simulink model "DBPSK_FormaEficiente"  (R2018b)
settings: Solver=ode5  StartTime=0.0  StopTime=(1/Rb)*CantSimb  FixedStep=(1/Rb)/1000  RelTol=1e-3
values from neighbouring files (symbols this model uses):
  Eb = EbPerf    [BDPSK.m]    (also in Codigo8DPSK.m; CodigoQDPSK.m)
  Fp = 10*Rb    [BDPSK.m]    (also in Codigo8DPSK.m; CodigoQDPSK.m)
  Rb = RbPerf    [BDPSK.m]    (also in Codigo8DPSK.m; CodigoQDPSK.m)
libraries: dspsigops x3, simulink x2, commchan3 x1, commrandsrc3 x1, commdigbbndpm3 x1
settings Model: Creator=lukit  LastModifiedBy=lukit

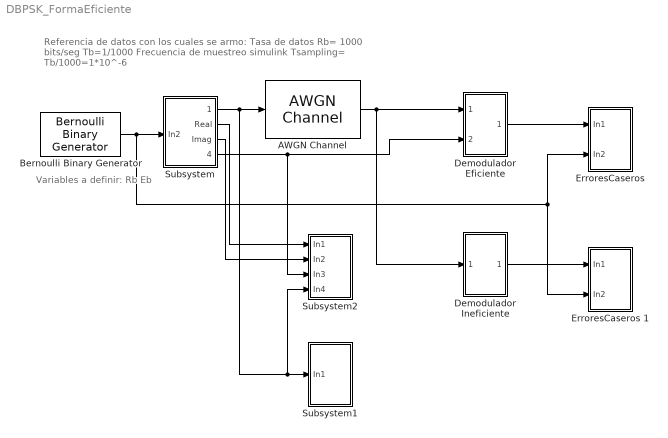
== system DBPSK_FormaEficiente ==
  note: Variables a definir:
      | Rb
      | Eb
  note: Referencia de datos con los cuales se armo:
      | Tasa de datos Rb= 1000 bits/seg Tb=1/1000
      | Frecuencia de muestreo simulink Tsampling= Tb/1000=1*10^-6
  AWGN Channel : commchan3/AWGN Channel  InputProcessing=Columns as channels (frame based)  seed=67  noiseMode="Signal to noise ratio  (Es/No)"  EbNodB=EsNo  EsNodB=EsNo  SNRdB=2  bitsPerSym=1  Ps=Eb/(1/Rb)  Tsym=(1/Rb)  variance=1
      settings: SourceProductName=Communications Toolbox
  Bernoulli Binary Generator : commrandsrc3/Bernoulli Binary Generator  ProbabilityOfZero=0.5  SeedSource=Auto  Seed=0  SampleTime=1/Rb  SamplesPerFrame=1  OutputDataType=double  SimulateUsing=Interpreted execution
      settings: SourceProductName=Communications Toolbox
  Demodulador Eficiente : Subsystem
  "Demodulador Ineficiente " : Subsystem
  "ErroresCaseros " : Subsystem
  ErroresCaseros 1 : Subsystem
  Subsystem : Subsystem
  Subsystem1 : Subsystem
  Subsystem2 : Subsystem
  wires:
  Bernoulli Binary Generator/1 -> ErroresCaseros 1/2(In2), "ErroresCaseros "/2(In2), Subsystem/1(In2)
  Subsystem/1(Salida) -> Subsystem2/4(In4), Subsystem1/1(In1), AWGN Channel/1
  Subsystem/4("Secuencia ") -> Subsystem2/3(In3), Demodulador Eficiente/2(In2)
  Demodulador Eficiente/1(Out1) -> "ErroresCaseros "/1(In1)
  AWGN Channel/1 -> "Demodulador Ineficiente "/1(In1), Demodulador Eficiente/1(In1)
  "Demodulador Ineficiente "/1(Out1) -> ErroresCaseros 1/1(In1)
  Subsystem/2(Real) -> Subsystem2/1(In1)
  Subsystem/3(Imag) -> Subsystem2/2(In2)

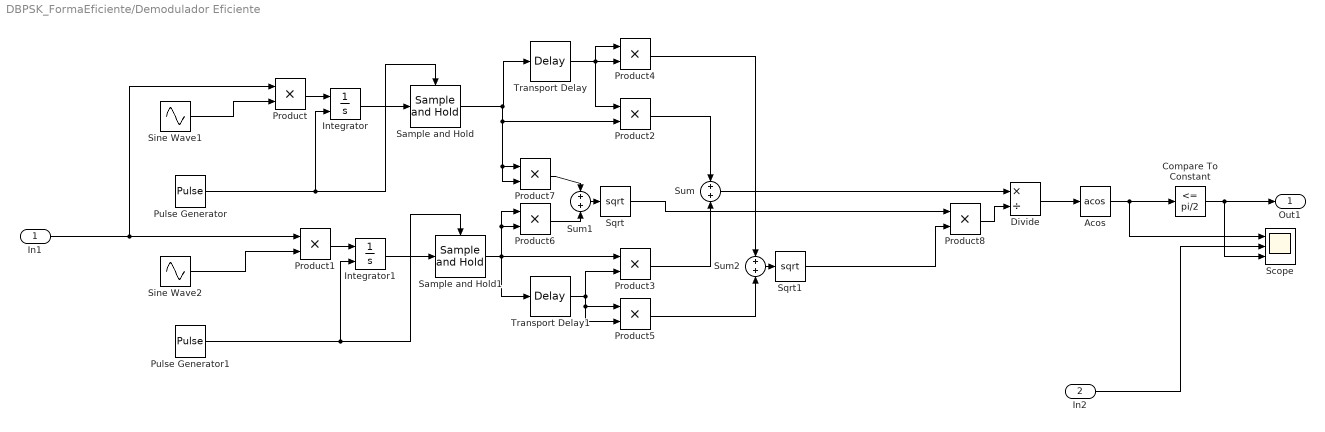
== system DBPSK_FormaEficiente/Demodulador Eficiente ==
  In1 : Inport
  In2 : Inport  Port=2
  Acos : Trigonometry  Operator=acos
  Compare To Constant : simulink/Logic and Bit Operations/Compare To Constant  relop=<=  const=pi/2  OutDataTypeStr=boolean
  Divide : Product  Inputs=*/
  Integrator : Integrator  ExternalReset=rising
  Integrator1 : Integrator  ExternalReset=rising
  Product{,1..8} (9 alike) : Product
  Pulse Generator : DiscretePulseGenerator  PulseType=Time based  Period=1/Rb  PulseWidth=99
  Pulse Generator1 : DiscretePulseGenerator  PulseType=Time based  Period=1/Rb  PulseWidth=99
  Sample and Hold : dspsigops/Sample and Hold  trig=Falling edge  initCond=0  latchinput=off
  Sample and Hold1 : dspsigops/Sample and Hold  trig=Falling edge  initCond=0  latchinput=off
  Scope : Scope  NumInputPorts=3
  Sine Wave1 : Sin  Amplitude=sqrt(2/(1/Rb))  Frequency=2*pi*Fp  Phase=pi/2
  Sine Wave2 : Sin  Amplitude=sqrt(2/(1/Rb))  Frequency=2*pi*Fp
  Sqrt : Sqrt  SaturateOnIntegerOverflow=on
  Sqrt1 : Sqrt  SaturateOnIntegerOverflow=on
  Sum : Sum
  Sum1 : Sum
  Sum2 : Sum
  Transport Delay : TransportDelay  DelayTime=1/Rb
  Transport Delay1 : TransportDelay  DelayTime=1/Rb
  Out1 : Outport
  wires:
  Integrator/1 -> Sample and Hold/1
  Pulse Generator/1 -> Sample and Hold/Trigger, Integrator/2
  Product/1 -> Integrator/1
  Integrator1/1 -> Sample and Hold1/1
  Product1/1 -> Integrator1/1
  Pulse Generator1/1 -> Sample and Hold1/Trigger, Integrator1/2
  Sample and Hold/1 -> Product7/2, Product7/1, Product2/2, Transport Delay/1
  Sample and Hold1/1 -> Product6/2, Product6/1, Transport Delay1/1, Product3/1
  Transport Delay1/1 -> Product5/2, Product5/1, Product3/2
  Transport Delay/1 -> Product4/1, Product4/2, Product2/1
  Product2/1 -> Sum/1
  Product3/1 -> Sum/2
  Product7/1 -> Sum1/1
  Product6/1 -> Sum1/2
  Sum1/1 -> Sqrt/1
  Product5/1 -> Sum2/2
  Product4/1 -> Sum2/1
  Sum2/1 -> Sqrt1/1
  Sum/1 -> Divide/1
  Product8/1 -> Divide/2
  Sqrt1/1 -> Product8/2
  Sqrt/1 -> Product8/1
  Divide/1 -> Acos/1
  Sine Wave1/1 -> Product/2
  Sine Wave2/1 -> Product1/2
  Acos/1 -> Compare To Constant/1, Scope/1
  In1/1 -> Product1/1, Product/1
  In2/1 -> Scope/2
  Compare To Constant/1 -> Scope/3, Out1/1

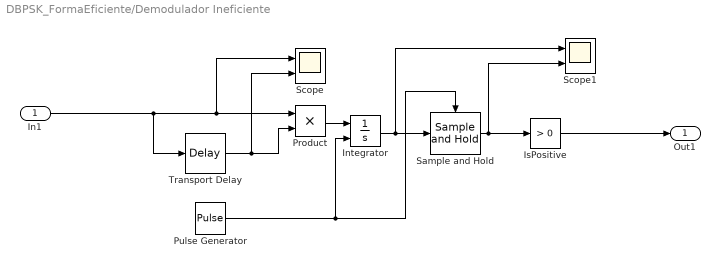
== system DBPSK_FormaEficiente/Demodulador Ineficiente  ==
  In1 : Inport
  Integrator : Integrator  ExternalReset=rising
  IsPositive : simulink/Logic and Bit Operations/Compare To Zero  relop=>  OutDataTypeStr=boolean
  Product : Product
  Pulse Generator : DiscretePulseGenerator  PulseType=Time based  Period=1/Rb  PulseWidth=99
  Sample and Hold : dspsigops/Sample and Hold  trig=Falling edge  initCond=0  latchinput=off
  Scope : Scope  NumInputPorts=2
  Scope1 : Scope  NumInputPorts=2
  Transport Delay : TransportDelay  DelayTime=(1/Rb)
  Out1 : Outport
  wires:
  Sample and Hold/1 -> Scope1/2, IsPositive/1
  In1/1 -> Transport Delay/1, Scope/1, Product/1
  Transport Delay/1 -> Product/2, Scope/2
  Integrator/1 -> Scope1/1, Sample and Hold/1
  Pulse Generator/1 -> Sample and Hold/Trigger, Integrator/2
  Product/1 -> Integrator/1
  IsPositive/1 -> Out1/1

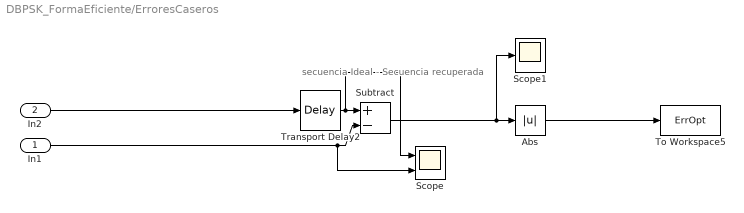
== system DBPSK_FormaEficiente/ErroresCaseros  ==
  note: secuencia Ideal - Secuencia recuperada
  In1 : Inport
  In2 : Inport  Port=2
  Abs : Abs
  Scope : Scope  NumInputPorts=2
  Scope1 : Scope
  Subtract : Sum  Inputs=+-
  To Workspace5 : ToWorkspace  VariableName=ErrOpt  SampleTime=-1
      settings: Save2DSignal=2-D array (concatenate along first dimension)
  Transport Delay2 : TransportDelay  DelayTime=(1/Rb)
  wires:
  Subtract/1 -> Scope1/1, Abs/1
  Transport Delay2/1 -> Scope/1, Subtract/1
  In1/1 -> Scope/2, Subtract/2
  In2/1 -> Transport Delay2/1
  Abs/1 -> To Workspace5/1

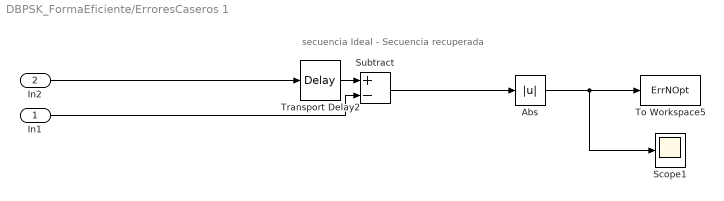
== system DBPSK_FormaEficiente/ErroresCaseros 1 ==
  note: secuencia Ideal - Secuencia recuperada
  In1 : Inport
  In2 : Inport  Port=2
  Abs : Abs
  Scope1 : Scope
  Subtract : Sum  Inputs=+-
  To Workspace5 : ToWorkspace  VariableName=ErrNOpt  SampleTime=-1
      settings: Save2DSignal=2-D array (concatenate along first dimension)
  Transport Delay2 : TransportDelay  DelayTime=(1/Rb)
  wires:
  Transport Delay2/1 -> Subtract/1
  In1/1 -> Subtract/2
  In2/1 -> Transport Delay2/1
  Subtract/1 -> Abs/1
  Abs/1 -> Scope1/1, To Workspace5/1

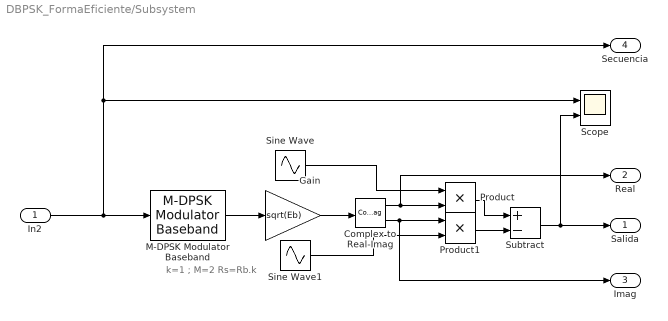
== system DBPSK_FormaEficiente/Subsystem ==
  note: k=1 ; M=2
      | Rs=Rb.k
  In2 : Inport
  Complex to Real-Imag : ComplexToRealImag
  Gain : Gain  Gain=sqrt(Eb)
  M-DPSK Modulator Baseband : commdigbbndpm3/M-DPSK Modulator Baseband  M=2  InType=Bit  Enc=Binary  Ph=pi  outDtype=double
      settings: SourceProductName=Communications Toolbox  SourceProductBaseCode=CM
  Product : Product
  Product1 : Product
  Scope : Scope  NumInputPorts=2
  Sine Wave : Sin  Amplitude=sqrt(2/(1/Rb))  Frequency=2*pi*Fp  Phase=pi/2
  Sine Wave1 : Sin  Amplitude=sqrt(2/(1/Rb))  Frequency=2*pi*Fp
  Subtract : Sum  Inputs=+-
  Salida : Outport
  Real : Outport  Port=2
  Imag : Outport  Port=3
  "Secuencia " : Outport  Port=4
  wires:
  Product/1 -> Subtract/1
  M-DPSK Modulator Baseband/1 -> Gain/1
  Sine Wave1/1 -> Product1/2
  Product1/1 -> Subtract/2
  Complex to Real-Imag/2 -> Imag/1, Product1/1
  Sine Wave/1 -> Product/1
  Complex to Real-Imag/1 -> Product/2, Real/1
  Subtract/1 -> Salida/1, Scope/2
  Gain/1 -> Complex to Real-Imag/1
  In2/1 -> M-DPSK Modulator Baseband/1, Scope/1, "Secuencia "/1

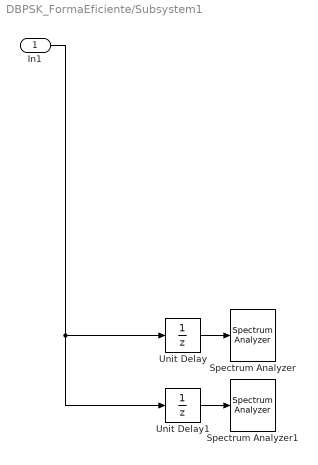
== system DBPSK_FormaEficiente/Subsystem1 ==
  In1 : Inport
  Spectrum Analyzer : SpectrumAnalyzer
  Spectrum Analyzer1 : SpectrumAnalyzer
  Unit Delay : UnitDelay  SampleTime=-1
  Unit Delay1 : UnitDelay  SampleTime=-1
  wires:
  In1/1 -> Unit Delay1/1, Unit Delay/1
  Unit Delay1/1 -> Spectrum Analyzer1/1
  Unit Delay/1 -> Spectrum Analyzer/1

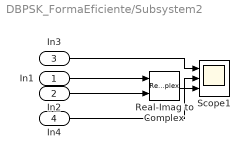
== system DBPSK_FormaEficiente/Subsystem2 ==
  In1 : Inport
  In2 : Inport  Port=2
  In3 : Inport  Port=3
  In4 : Inport  Port=4
  Real-Imag to Complex : RealImagToComplex
  Scope1 : Scope  NumInputPorts=3
  wires:
  In3/1 -> Scope1/1
  Real-Imag to Complex/1 -> Scope1/3
  In1/1 -> Real-Imag to Complex/1
  In4/1 -> Scope1/2
  In2/1 -> Real-Imag to Complex/2
